simulink model "q1"  (R2016a)
settings: Solver=VariableStepAuto  StartTime=0.0  StopTime=10.0  RelTol=1e-3
settings Model: Creator=cinlab  LastModifiedBy=cinlab

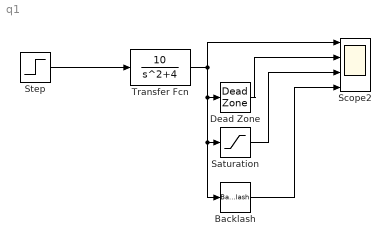
== system q1 ==
  Backlash : Backlash  BacklashWidth=2
  Dead Zone : DeadZone  LowerValue=-2  UpperValue=2  SaturateOnIntegerOverflow=on
  Saturation : Saturate  UpperLimit=2  LowerLimit=-2
  Scope2 : Scope  NumInputPorts=4
  Step : Step  Time=0  SampleTime=0
  Transfer Fcn : TransferFcn  Numerator=[10]  Denominator=[1 0 4]
  wires:
  Step/1 -> Transfer Fcn/1
  Saturation/1 -> Scope2/3
  Transfer Fcn/1 -> Dead Zone/1, Backlash/1, Saturation/1, Scope2/1
  Backlash/1 -> Scope2/4
  Dead Zone/1 -> Scope2/2
